simulink model "rectufyingcircuit"  (R2018a)
settings: Solver=ode4  StartTime=0.0  StopTime=50  FixedStep=0.01  RelTol=1e-3
undefined symbols (not defined in the file): Imag, Real
libraries: powerlib x14
settings Model: Creator=lenovo  LastModifiedBy=lenovo

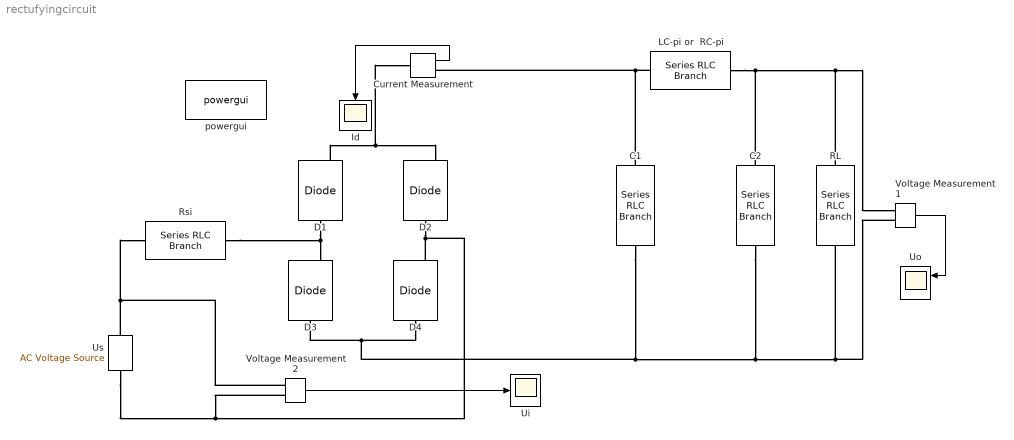
== system rectufyingcircuit ==
  C1 : powerlib/Elements/Series RLC Branch  LConnTagsString=__new0  RConnTagsString=__new0  BranchType=C  Resistance=10000000  Inductance=0  SetiL0=off  InitialCurrent=0  Capacitance=0.0085  Setx0=off  InitialVoltage=0  Measurements=None
  C2 : powerlib/Elements/Series RLC Branch  LConnTagsString=__new0  RConnTagsString=__new0  BranchType=C  Resistance=1000000  Inductance=0  SetiL0=off  InitialCurrent=0  Capacitance=0.00942  Setx0=off  InitialVoltage=0  Measurements=None
  Current Measurement : powerlib/Measurements/Current Measurement  PhasorSimulation=off  OutputType=Real-Imag  PSBequivalent=0
  D{1..4} (4 alike) : powerlib/Power Electronics/Diode  Ron=0  Lon=0  Vf=0.7  IC=0  UseSnubber=0  Rs=5000000000  Cs=0  Measurements=on
  Id : Scope
  LC-pi or  RC-pi : powerlib/Elements/Series RLC Branch  LConnTagsString=__new0  RConnTagsString=__new0  BranchType=RL  Resistance=50  Inductance=0  SetiL0=off  InitialCurrent=0  Capacitance=0  Setx0=off  InitialVoltage=0  Measurements=None
  RL : powerlib/Elements/Series RLC Branch  LConnTagsString=__new0  RConnTagsString=__new0  BranchType=R  Resistance=1000  Inductance=0  SetiL0=off  InitialCurrent=0  Capacitance=0  Setx0=off  InitialVoltage=0  Measurements=None
  Rsi : powerlib/Elements/Series RLC Branch  LConnTagsString=__new0  RConnTagsString=__new0  BranchType=R  Resistance=1  Inductance=0  SetiL0=off  InitialCurrent=0  Capacitance=0  Setx0=off  InitialVoltage=0  Measurements=None
  Ui : Scope
  Uo : Scope  NumInputPorts=2
  Us : powerlib/Electrical Sources/AC Voltage Source  Amplitude=1000  Phase=0  Frequency=0.6  SampleTime=0  Measurements=None  BusType=swing  Pref=10e3  Qref=0  Qmin=-inf  Qmax=+inf
  Voltage Measurement1 : powerlib/Measurements/Voltage Measurement  PhasorSimulation=off  OutputType=Real-Imag  PSBequivalent=0
  Voltage Measurement2 : powerlib/Measurements/Voltage Measurement  PhasorSimulation=off  OutputType=Real-Imag  PSBequivalent=0
  powergui : powerlib/powergui  Priority=1  SimulationMode=Continuous  SampleTime=50e-6  frequency=60  Iterations=50  frequencyindice=0  Pbase=100e6  ErrMax=1e-4  UnitsV=kV  UnitsW=MW  buscounter=0  FunctionMessages=off  echomessages=off  EnableUseOfTLC=off  CurrentSourceSwitches=off  DisableSnubberDevices=off  DisableRonSwitches=off  DisableVfSwitches=off  DisplayEquations=off  SolverType=Tustin/Backward Euler (TBE)  Interpol=off  ExternalGateDelay=off  methode=off  Ts=100  x0status=blocks  SPID=off  SwTol=0  HookPort=off  RestoreLinks=warning  ResistiveCurrentMeasurement=off  Frange=[0:2:500]  Ylog=off  Xlog=on  ShowGrid=off  save=off  variable=ZData  structure=0  ZoomFFT=off  StartTime=0.0  cycles=1  DisplayStyle=1  fundamental=60  FreqAxis=off  MaxFrequency=1000  frequencyindicesteady=1  RmsSteady=1  display=off
  wires:
  Voltage Measurement1/1 -> Uo/1
  Current Measurement/1 -> Id/1
  Voltage Measurement2/1 -> Ui/1
  connections:
  D2/LConn1 -- Us/LConn1 -- Voltage Measurement2/LConn2 -- D4/RConn1
  Voltage Measurement1/LConn2 -- C1/RConn1 -- D4/LConn1 -- D3/LConn1 -- C2/RConn1 -- RL/RConn1
  Us/RConn1 -- Voltage Measurement2/LConn1 -- Rsi/RConn1
  D1/RConn1 -- Current Measurement/LConn1 -- D2/RConn1
  Rsi/LConn1 -- D1/LConn1 -- D3/RConn1
  LC-pi or  RC-pi/LConn1 -- RL/LConn1 -- Voltage Measurement1/LConn1 -- C2/LConn1
  LC-pi or  RC-pi/RConn1 -- C1/LConn1 -- Current Measurement/RConn1
